simulink model "q1e_attempt_3"  (R2021b)
settings: Solver=VariableStepAuto  StartTime=0.0  StopTime=16  RelTol=1e-3
undefined symbols (not defined in the file or in its folder): sigbuilder_block
libraries: simulink_extras x1
settings Model: Creator=joero  LastModifiedBy=joero

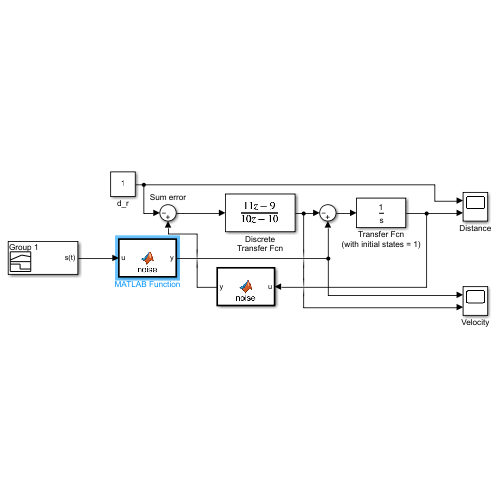
[thumbnail: Simulink's stored preview of the top-level diagram]
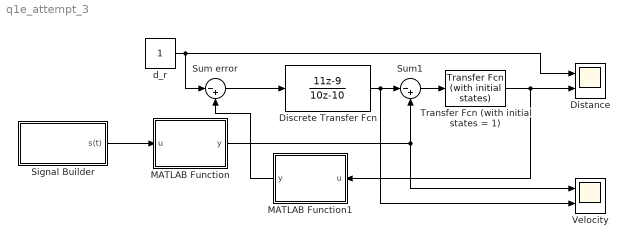
== system q1e_attempt_3 ==
  Discrete Transfer Fcn : DiscreteTransferFcn  Numerator=[11 -9]  Denominator=[10 -10]  InitialStates=1
  Distance : Scope  NumInputPorts=2
  MATLAB Function : MATLAB Function  TreatAsAtomicUnit=on
  MATLAB Function1 : MATLAB Function  TreatAsAtomicUnit=on
  Signal Builder : Subsystem  Tag=STV Subsys  LoadFcn=sigbuilder_block('load');  StartFcn=sigbuilder_block('start');  StopFcn=sigbuilder_block('stop');  ClipboardFcn=sigbuilder_block('clipboard');  mask(Sigbuilder block){tuvar=[0:10]}
      mask help: Simulink:masks:SigbuilderBlock_MD
      mask init:
      | if ~strcmp(get_param(bdroot(gcbh),'SimulationStatus'),'stopped') tuvar = sigbuilder_block('maskInit'); end
      settings: CopyFcn=sigbuilder_block('copy');  DeleteFcn=sigbuilder_block('delete');  ModelCloseFcn=sigbuilder_block('modelClose');  PreSaveFcn=sigbuilder_block('preSave');  PauseFcn=sigbuilder_block('pause');  ContinueFcn=sigbuilder_block('continue');  NameChangeFcn=sigbuilder_block('namechange');  OpenFcn=sigbuilder_block('open',[4.5 30 951 425.25 ]);  CloseFcn=sigbuilder_block('close');
      mask Display: plot(0, 0, 100, 100,[2, 2, 32, 32, 2], [68, 8, 8, 68, 68],[32, 2], [38, 38], [32, 19, 2],[53, 60, 44], [32, 17, 17, 2],[16, 16, 31, 31]);txt = getActiveGroup(gcbh);text(2, 100, txt,'verticalAlignment', 'top');
  Sum error : Sum  Inputs=|-+
  Sum1 : Sum  Inputs=|-+
  Transfer Fcn (with initial states = 1) : simulink_extras/Additional Linear/Transfer Fcn (with initial states)  N=[1]  D="[1  0]"  X0=0
  Velocity : Scope  NumInputPorts=2
  d_r : Constant
  wires:
  Signal Builder/1(s(t)) -> MATLAB Function/1(u)
  Transfer Fcn (with initial states = 1)/1 -> MATLAB Function1/1(u), Distance/2
  MATLAB Function/1(y) -> Sum1/2, Velocity/1
  Sum1/1 -> Transfer Fcn (with initial states = 1)/1
  d_r/1 -> Distance/1, Sum error/1
  Discrete Transfer Fcn/1 -> Sum1/1, Velocity/2
  MATLAB Function1/1(y) -> Sum error/2
  Sum error/1 -> Discrete Transfer Fcn/1

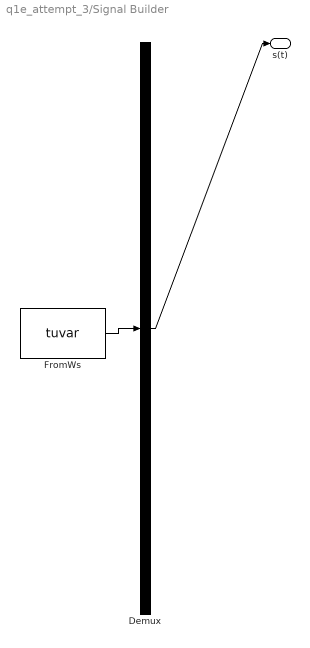
== system q1e_attempt_3/Signal Builder ==
  Demux : Demux  Tag=STV Demux  Outputs=1
      settings: DisplayOption=none
  FromWs : FromWorkspace  Tag=STV FromWs  VariableName=tuvar
      SigBuilderData=|
      | common.afterFinalStr = 'Extrapolate'
      | common.sampleTime = 0
      | dataSet.timeRange = [0 16]
      | dataSet.name = 'Group 1'
      | sbobj.Groups.Name = 'Group 1'
      | sbobj.Groups.Signals.Name = 's(t)'
      | sbobj.Groups.Signals.XData = [0 4 8 10 16]
      | sbobj.Groups.Signals.YData = [0 0.4 0.4 0.2 0.2]
      | sbobj.Groups.TimeRange = [0 16]
  s(t) : Outport  Tag=STV Outport
  wires:
  FromWs/1 -> Demux/1
  Demux/1 -> s(t)/1

== matlab function q1e_attempt_3/MATLAB Function ==
  settings: updateMethod=DISCRETE
  data: u input; y output
function y = noise(u)
mean = 0;
standard_dev = 0.01;
y = u + standard_dev*randn(1)+ mean;

== matlab function q1e_attempt_3/MATLAB Function1 ==
  settings: updateMethod=DISCRETE
  data: u input; y output
function y = noise(u)
% std = sqrt(var)
mean = 0;
standard_dev = 0.01;
y = u + standard_dev*randn(1)+ mean;
